simulink model "example"  (R2013a)
settings: Solver=ode45  StartTime=0.0  StopTime=10.0  RelTol=1e-3
values from neighbouring files (symbols this model uses):
  Jmotor = 1.9e-3    (= 0.0019)    [act_damp_var.m]    (also in act_damp_var_Linmod.m)
  Ka = 2.284    [act_damp_var.m]    (also in act_damp_var_Linmod.m)
  Kb = 2.284    [act_damp_var.m]    (also in act_damp_var_Linmod.m)
  Kphi = 4.9e-3    (= 0.0049)    [act_damp_var.m]    (also in act_damp_var_Linmod.m)
  Kt = 2.0336e5    (= 203360)    [act_damp_var.m]    (also in act_damp_var_Linmod.m)
  La = 9.05e-4    (= 0.000905)    [act_damp_var.m]    (also in act_damp_var_Linmod.m)
  ma = 1    [act_damp_var.m]    (also in act_damp_var_Linmod.m)
  mb = 1    [act_damp_var.m]    (also in act_damp_var_Linmod.m)
  mc = 1    [act_damp_var.m]    (also in act_damp_var_Linmod.m)
  rp = 0.75    [act_damp_var.m]    (also in act_damp_var_Linmod.m)
  Rt = 1    [act_damp_var_Linmod.m]
  SampTime = 0.02    [act_damp_var.m]    (also in act_damp_var_Linmod.m)
settings Model: Creator=Jon's-Laptop  LastModifiedBy=Jon's-Laptop

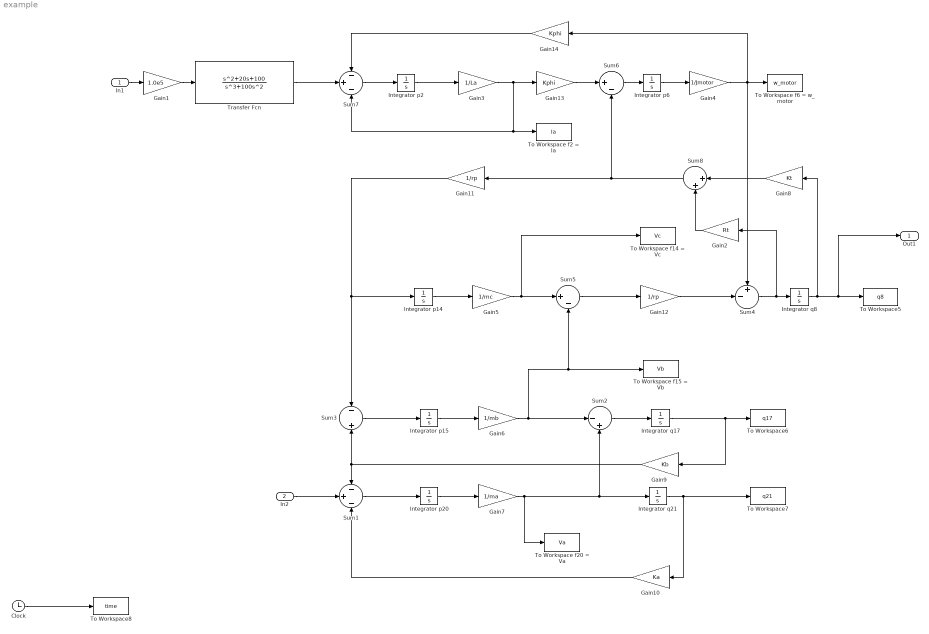
== system example ==
  In1 : Inport
  In2 : Inport  Port=2
  Clock : Clock
  Gain1 : Gain  Gain=1.0e5
  Gain10 : Gain  Gain=Ka
  Gain11 : Gain  Gain=1/rp
  Gain12 : Gain  Gain=1/rp
  Gain13 : Gain  Gain=Kphi
  Gain14 : Gain  Gain=Kphi
  Gain2 : Gain  Gain=Rt
  Gain3 : Gain  Gain=1/La
  Gain4 : Gain  Gain=1/Jmotor
  Gain5 : Gain  Gain=1/mc
  Gain6 : Gain  Gain=1/mb
  Gain7 : Gain  Gain=1/ma
  Gain8 : Gain  Gain=Kt
  Gain9 : Gain  Gain=Kb
  Integrator p{2,6,14..15,20} (5 alike) : Integrator
  Integrator q17 : Integrator
  Integrator q21 : Integrator
  Integrator q8 : Integrator
  Sum1 : Sum  Inputs=-+-
  Sum2 : Sum  Inputs=|-+
  Sum3 : Sum  Inputs=-|+
  Sum4 : Sum  Inputs=+-|
  Sum5 : Sum  Inputs=|+-
  Sum6 : Sum  Inputs=|+-
  Sum7 : Sum  Inputs=-+-
  Sum8 : Sum  Inputs=|++
  To Workspace f14 = Vc : ToWorkspace  VariableName=Vc  SampleTime=SampTime
  To Workspace f15 = Vb : ToWorkspace  VariableName=Vb  SampleTime=SampTime
  To Workspace f2 = Ia : ToWorkspace  VariableName=Ia  SampleTime=SampTime
  To Workspace f20 = Va : ToWorkspace  VariableName=Va  SampleTime=SampTime
  To Workspace f6 = w_motor : ToWorkspace  VariableName=w_motor  SampleTime=SampTime
  To Workspace5 : ToWorkspace  VariableName=q8  SampleTime=SampTime
  To Workspace6 : ToWorkspace  VariableName=q17  SampleTime=SampTime
  To Workspace7 : ToWorkspace  VariableName=q21  SampleTime=SampTime
  To Workspace8 : ToWorkspace  VariableName=time  SampleTime=SampTime
  Transfer Fcn : TransferFcn  Numerator=[1 20 100]  Denominator=[1 100 0 0]
  Out1 : Outport
  wires:
  Clock/1 -> To Workspace8/1
  Integrator q8/1 -> Gain8/1, Out1/1, To Workspace5/1
  Integrator q17/1 -> Gain9/1, To Workspace6/1
  Integrator q21/1 -> Gain10/1, To Workspace7/1
  Integrator p2/1 -> Gain3/1
  Gain3/1 -> To Workspace f2 = Ia/1, Sum7/3, Gain13/1
  Integrator p6/1 -> Gain4/1
  Gain4/1 -> To Workspace f6 = w_motor/1, Sum4/1, Gain14/1
  Integrator p14/1 -> Gain5/1
  Gain5/1 -> To Workspace f14 = Vc/1, Sum5/1
  Integrator p15/1 -> Gain6/1
  Gain6/1 -> Sum2/1, To Workspace f15 = Vb/1, Sum5/2
  Integrator p20/1 -> Gain7/1
  Gain7/1 -> Integrator q21/1, Sum2/2, To Workspace f20 = Va/1
  Sum1/1 -> Integrator p20/1
  Gain10/1 -> Sum1/3
  Gain9/1 -> Sum3/2, Sum1/1
  Sum2/1 -> Integrator q17/1
  Sum3/1 -> Integrator p15/1
  Gain11/1 -> Sum3/1, Integrator p14/1
  Sum4/1 -> Gain2/1, Integrator q8/1
  Gain12/1 -> Sum4/2
  Sum5/1 -> Gain12/1
  Sum6/1 -> Integrator p6/1
  Gain13/1 -> Sum6/1
  Gain14/1 -> Sum7/1
  Sum7/1 -> Integrator p2/1
  In2/1 -> Sum1/2
  In1/1 -> Gain1/1
  Transfer Fcn/1 -> Sum7/2
  Gain1/1 -> Transfer Fcn/1
  Gain8/1 -> Sum8/1
  Sum8/1 -> Sum6/2, Gain11/1
  Gain2/1 -> Sum8/2
